simulink model "sim_test"  (R2016b)
settings: Solver=ode3  StartTime=0.0  StopTime=Tsim  FixedStep=Ts  RelTol=1e-3  EnableMultiTasking=on
InitFcn:
  | load('dyn_param.mat')
values from neighbouring files (symbols this model uses):
  C_meas = -[zeros(ny,3) eye(ny)]    [run_comparison.m]
  C_scope = [eye(2) zeros(2,1+ny)]    [run_comparison.m]
  dist = 2e-2    (= 0.02)    [run_comparison.m]
  gamm = 0    [dyn_param.mat]
  P = ss(A,[Bw Bu],[Cz;Cy],[Dzw Dzu; Dyw zeros(size(Cy,1),1)])    [system_def.m]
  ref = 1    [run_comparison.m]
  Tdist = 15    [run_comparison.m]
  Tref = 2    [run_comparison.m]
  x0 = [0;zeros(size(P.A,1)-1,1)]    [run_comparison.m]
undefined symbols (not defined in the file or in its folder): Ksys, xK0
settings Model: Creator=Matti  LastModifiedBy=user
settings OptimizationCC: LifeSpan=inf
settings DebuggingCC: SFUnexpectedBacktrackingDiag=warning  SFNoUnconditionalDefaultTransitionDiag=warning  SFExecutionAtInitializationDiag=none
settings GRTTargetCC: TargetLangStandard=C89/C90 (ANSI)  GeneratePreprocessorConditionals=Disable all
settings ConfigComp: CovMetricSettings=dw  CovHtmlReporting=on  CovSaveCumulativeToWorkspaceVar=on  CovSaveSingleToWorkspaceVar=on  CovExternalEMLEnable=off

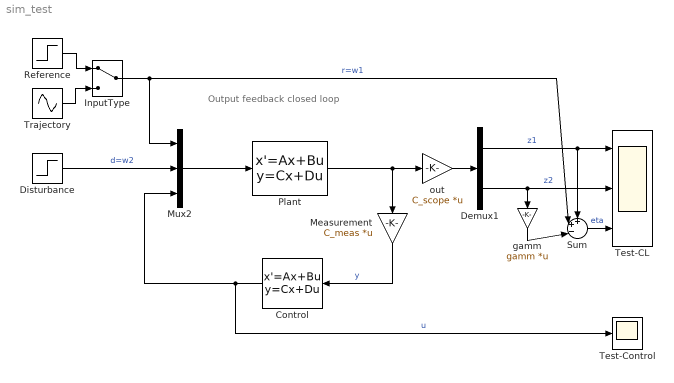
== system sim_test ==
  note: Output feedback closed loop
  Control : StateSpace  A=Ksys.A  B=Ksys.B  C=Ksys.C  D=Ksys.D  X0=xK0
  Demux1 : Demux  Outputs=2
  Disturbance : Step  Time=Tdist  After=dist  SampleTime=0
  InputType : ManualSwitch
  Measurement : Gain  Gain=C_meas  Multiplication=Matrix(K*u)
  Mux2 : Mux  Inputs=3
  Plant : StateSpace  A=P.A  B=P.B  C=P.C  D=P.D  X0=x0
  Reference : Step  Time=Tref  After=ref  SampleTime=0
  Sum : Sum  Inputs=++-|
  Test-CL : Scope  NumInputPorts=3
  Test-Control : Scope
  Trajectory : Sin  Frequency=0.5  SampleTime=0
  gamm : Gain  Gain=gamm  Multiplication=Matrix(K*u)
  out : Gain  Gain=C_scope  Multiplication=Matrix(K*u)
  wires:
  Disturbance/1 -> Mux2/2  "d=w2"
  Measurement/1 -> Control/1  "y"
  Plant/1 -> Measurement/1, out/1
  Control/1 -> Test-Control/1, Mux2/3  "u"
  Mux2/1 -> Plant/1
  Reference/1 -> InputType/1
  InputType/1 -> Sum/2, Mux2/1  "r=w1"
  Trajectory/1 -> InputType/2
  Demux1/1 -> Sum/1, Test-CL/1  "z1"
  out/1 -> Demux1/1
  Demux1/2 -> gamm/1, Test-CL/2  "z2"
  Sum/1 -> Test-CL/3  "eta"
  gamm/1 -> Sum/3
